simulink model "servo_model_v1"  (R2016a)
settings: Solver=VariableStepAuto  StartTime=0.0  StopTime=15  RelTol=1e-3
libraries: powerlib x4
settings Model: Creator=user  LastModifiedBy=user

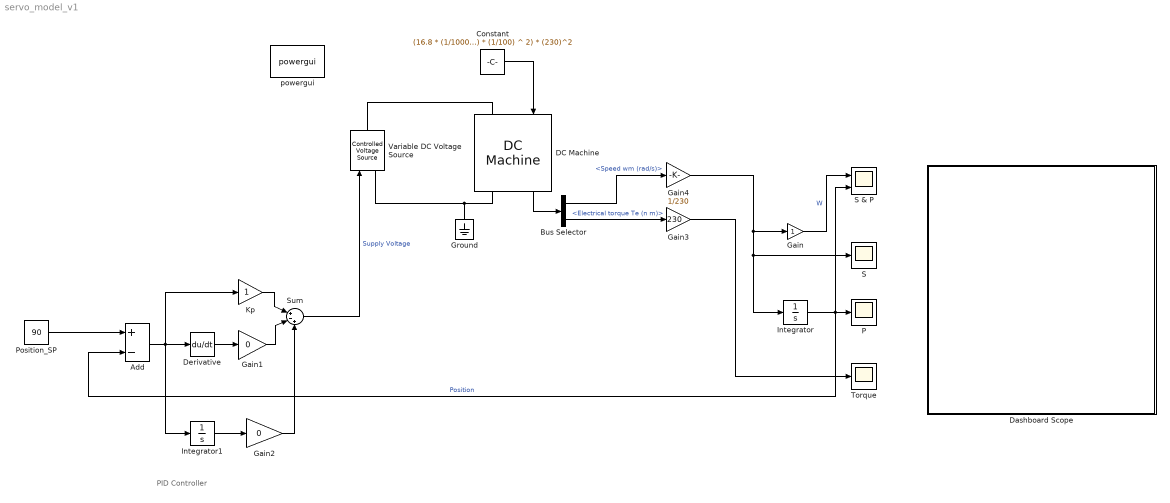
== system servo_model_v1 ==
  note: PID Controller
  Add : Sum  Inputs=+-
  Bus Selector : BusSelector  OutputSignals=Speed wm (rad/s),Electrical torque Te (n m)
  Constant : Constant  Value=(16.8 * (1/1000) * (1/100) ^ 2) * (230)^2
  DC Machine : powerlib/Machines/DC Machine  PresetModel=No  MechanicalLoad=Torque TL  FieldType=Permanent magnet  ShowDetailedParameters=on  MeasurementBus=off  RLa="[ 0.299  0.082e-3]"  RLf="[ 240  120]"  Laf=1.8  MachineConstant=Back-emf constant (V/rpm)  Ke=1/317  Kt=30.2/1000  J=142 * (1/1000) * (1/100) ^ 2  Bm=0  Tf=0  w0=2  Ifinit=2  TsPowergui=0  TsBlock=-1
  Dashboard Scope : Subsystem  DialogController=hmiCreateDDGDialog  IsWebBlock=on  mask(MWDashboardBlock){webBlockId=e0393ac5-2a71-4ae0-bf33-b12112959aa6, webBlockType=sdiscope, ShowInitialText=on, HMISrcModelName=servo_model_v1}
      mask prompts: webBlockId "WebBlock Id"; webBlockType "WebBlock Type"; HMISrcModelName "Source Model"
      mask Help: helpview([docroot '/mapfiles/simulink.map'], 'hmi_scope')
      mask Display:
      | if strcmp(get_param(bdroot(gcb),'BlockDiagramType'), 'library')
      |     image([(matlabroot) '/toolbox/simulink/hmi/icons/DashboardScope.png']);
      | end
  Derivative : Derivative
  Gain : Gain
  Gain1 : Gain  Gain=0
  Gain2 : Gain  Gain=0
  Gain3 : Gain  Gain=230
  Gain4 : Gain  Gain=1/230
  Ground : powerlib/Elements/Ground  LConnTagsString=a
  Integrator : Integrator
  Integrator1 : Integrator  InitialCondition=100
  Kp : Gain
  P : Scope
  Position_SP : Constant  Value=90
  S : Scope
  S & P : Scope  NumInputPorts=2
  Sum : Sum  Inputs=|+-+
  Torque : Scope
  Variable DC Voltage Source : powerlib/Electrical Sources/Controlled Voltage Source  Initialize=on  Source_Type=DC  Amplitude=0  Phase=0  Frequency=0  Measurements=Voltage
  powergui : powerlib/powergui  Priority=1  SimulationMode=Continuous  SolverType=Tustin/Backward Euler (TBE)  SampleTime=50e-6  frequency=60  SPID=off  DisableSnubberDevices=off  DisableRonSwitches=off  DisableVfSwitches=off  SwTol=0  DisplayEquations=off  Interpol=off  ExternalGateDelay=off  methode=off  Ts=10  FunctionMessages=off  echomessages=off  HookPort=off  EnableUseOfTLC=off  x0status=blocks  frequencyindice=0  Pbase=100e6  ErrMax=1e-4  Iterations=50  UnitsV=kV  UnitsW=MW  buscounter=0  RestoreLinks=warning  ResistiveCurrentMeasurement=off  Frange=[0:2:500]  Ylog=off  Xlog=on  ShowGrid=off  save=off  variable=ZData  structure=0  ZoomFFT=off  StartTime=0.0  cycles=1  DisplayStyle=1  fundamental=60  FreqAxis=off  MaxFrequency=1000  frequencyindicesteady=1  RmsSteady=1  display=off
  wires:
  Constant/1 -> DC Machine/1
  DC Machine/1 -> Bus Selector/1
  Integrator/1 -> Add/2, P/1, S & P/2  "Position"
  Gain/1 -> S & P/1  "W"
  Position_SP/1 -> Add/1
  Add/1 -> Integrator1/1, Derivative/1, Kp/1
  Derivative/1 -> Gain1/1
  Kp/1 -> Sum/1
  Gain1/1 -> Sum/2
  Sum/1 -> Variable DC Voltage Source/1  "Supply Voltage"
  Integrator1/1 -> Gain2/1
  Gain2/1 -> Sum/3
  Bus Selector/2 -> Gain3/1  "<Electrical torque Te (n m)>"
  Gain3/1 -> Torque/1
  Bus Selector/1 -> Gain4/1  "<Speed wm (rad/s)>"
  Gain4/1 -> Gain/1, S/1, Integrator/1
  connections:
  Ground/LConn1 -- Variable DC Voltage Source/LConn1 -- DC Machine/RConn1
  DC Machine/LConn1 -- Variable DC Voltage Source/RConn1

== system servo_model_v1/Dashboard Scope ==
